simulink library "IO"  (R2024a)
settings: Solver=VariableStepAuto  StartTime=0.0  StopTime=10.0  RelTol=1e-3
values from neighbouring files (symbols this model uses):
  ADCBits = 12.0    [IO.sldd]
  DigitalPolarity : value not decoded    [IO.sldd]
  Vref = 5.0    [IO.sldd]
undefined symbols (not defined in the file or in its folder): Bridge, dt, enum2Raptor, H, raptor_xcp_function
libraries: Raptor_lib x118, Utilities x27, Cooling x1
(part 2 of 4)

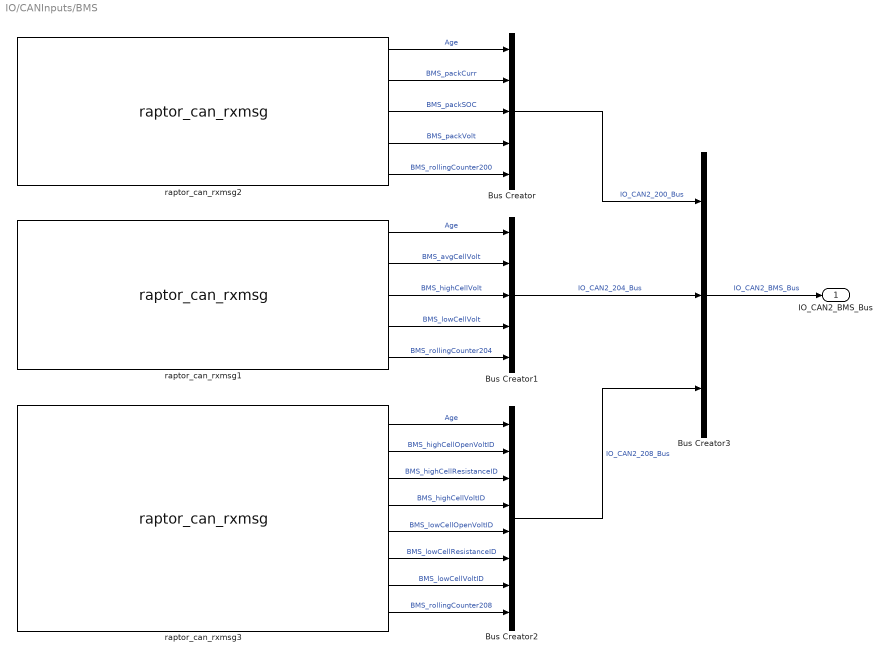
== system IO/CANInputs/BMS ==
  Bus Creator : BusCreator  Inputs=5
  Bus Creator1 : BusCreator  Inputs=5
  Bus Creator2 : BusCreator  Inputs=8
  Bus Creator3 : BusCreator  Inputs=3
  raptor_can_rxmsg1 : Raptor_lib/CAN/raptor_can_rxmsg  canDefinition=struct('dbcFile', 'raptor_CAN2.dbc','message', 'BMS_204','comment', '','signals', {{'BMS_avgCellVolt','BMS_highCellVolt','BMS_lowCellVolt','BMS_rollingCounter204'}},'enabled', [ 1 1 1 1;],'scaled', [ 1 1 1 1;],'canBus', '''CAN2''','messageID', [ 204;],'idMask', [ 536870911;],'payloadMask', [],'payloadValue', [],'period', [ 0;],'mailbox', '''''','queueSize', [ 1;],'label', [ 1;],'ver', [ 2;],'showID', [ 0;],'showRaw', [ 0;],'showRawMsg', [ 0;],'useStartVals', [ 0;],'extendedId', [ 0;],'showAge', [ 1;],'useSimFunc', [ 0;],'sim_func_name', '''''','fill', [ 0;],'editID', [ 0;],'signalOrder', [ 1;],'signalAscDes', [ 1;],'msgLength', [ 8;])  canBus='CAN2'  mailbox=''  payloadMask=[]  payloadValue=[]  idMask=hex2dec('1FFFFFFF')  queueSize=1  showID=0  label=1  fill=0  id=204  showRaw=0  showAge=1  signalOrder=1  signalInfo={{struct('Name', 'BMS_rollingCounter204','StartBit', [ 0;],'SignalSize', [ 8;],'ByteOrder', 'LittleEndian','ValueType', 'UNSIGNED','Class', 'uint8','Signed', [ 0;],'Factor', [ 1;],'Offset', [ 0;],'Min', [ 0;],'Max', [ 255;],'Units', '','StartVal', [ 0;],'Comment', 'Increments once every 100ms (max value is 255 and rolls over). Can be used to ensure data is updating','Multiplexed', [ 0;],'Multiplexor', [ 0;],'MultiplexMode_Min', [],'MultiplexMode_Max', []),struct('Name', 'BMS_lowCellVolt','StartBit', [ 16;],'SignalSize', [ 16;],'ByteOrder', 'LittleEndian','ValueType', 'SIGNED','Class', 'int16','Signed', [ 1;],'Factor', [ 0.0001;],'Offset', [ 0;],'Min', [ -3.2768;],'Max', [ 3.2767;],'Units', 'V','StartVal', [ 0;],'Comment', 'This is the voltage of the lowest measured cell in the battery pack','Multiplexed', [ 0;],'Multiplexor', [ 0;],'MultiplexMode_Min', [],'MultiplexMode_Max', []),struct('Name', 'BMS_highCellVolt','StartBit', [ 32;],'SignalSize', [ 16;],'ByteOrder', 'LittleEndian','ValueType', 'SIGNED','Class', 'int16','Signed', [ 1;],'Factor', [ 0.0001;],'Offset', [ 0;],'Min', [ -3.2768;],'Max', [ 3.2767;],'Units', 'V','StartVal', [ 0;],'Comment', 'This is the voltage of the highest measured cell in the battery pack','Multiplexed', [ 0;],'Multiplexor', [ 0;],'MultiplexMode_Min', [],'MultiplexMode_Max', []),struct('Name', 'BMS_avgCellVolt','StartBit', [ 48;],'SignalSize', [ 16;],'ByteOrder', 'LittleEndian','ValueType', 'SIGNED','Class', 'int16','Signed', [ 1;],'Factor', [ 0.0001;],'Offset', [ 0;],'Min', [ -3.2768;],'Max', [ 3.2767;],'Units', 'V','StartVal', [ 0;],'Comment', 'This is the voltage of the average measured cell in the battery pack','Multiplexed', [ 0;],'Multiplexor', [ 0;],'MultiplexMode_Min', [],'MultiplexMode_Max', [])}}  showRawMsg=0  useSimFunc=0  sim_func_name=''  useStartVals=0  extendedId=0
      settings: SourceProductName=Raptor
  raptor_can_rxmsg2 : Raptor_lib/CAN/raptor_can_rxmsg  canDefinition=struct('dbcFile', 'raptor_CAN2.dbc','message', 'BMS_200','comment', '','signals', {{'BMS_packCurr','BMS_packSOC','BMS_packVolt','BMS_rollingCounter200'}},'enabled', [ 1 1 1 1;],'scaled', [ 1 1 1 1;],'canBus', '''CAN2''','messageID', [ 200;],'idMask', [ 536870911;],'payloadMask', [],'payloadValue', [],'period', [ 0;],'mailbox', '''''','queueSize', [ 1;],'label', [ 1;],'ver', [ 2;],'showID', [ 0;],'showRaw', [ 0;],'showRawMsg', [ 0;],'useStartVals', [ 0;],'extendedId', [ 0;],'showAge', [ 1;],'useSimFunc', [ 0;],'sim_func_name', '''''','fill', [ 0;],'editID', [ 0;],'signalOrder', [ 1;],'signalAscDes', [ 1;],'msgLength', [ 8;])  canBus='CAN2'  mailbox=''  payloadMask=[]  payloadValue=[]  idMask=hex2dec('1FFFFFFF')  queueSize=1  showID=0  label=1  fill=0  id=200  showRaw=0  showAge=1  signalOrder=1  signalInfo={{struct('Name', 'BMS_rollingCounter200','StartBit', [ 0;],'SignalSize', [ 8;],'ByteOrder', 'LittleEndian','ValueType', 'UNSIGNED','Class', 'uint8','Signed', [ 0;],'Factor', [ 1;],'Offset', [ 0;],'Min', [ 0;],'Max', [ 255;],'Units', '','StartVal', [ 0;],'Comment', 'Increments once every 100ms (max value is 255 and rolls over). Can be used to ensure data is updating','Multiplexed', [ 0;],'Multiplexor', [ 0;],'MultiplexMode_Min', [],'MultiplexMode_Max', []),struct('Name', 'BMS_packVolt','StartBit', [ 32;],'SignalSize', [ 16;],'ByteOrder', 'LittleEndian','ValueType', 'SIGNED','Class', 'int16','Signed', [ 1;],'Factor', [ 0.1;],'Offset', [ 0;],'Min', [ -3276.8;],'Max', [ 3276.7;],'Units', 'V','StartVal', [ 0;],'Comment', 'This is the instantaneous total pack voltage value','Multiplexed', [ 0;],'Multiplexor', [ 0;],'MultiplexMode_Min', [],'MultiplexMode_Max', []),struct('Name', 'BMS_packSOC','StartBit', [ 48;],'SignalSize', [ 8;],'ByteOrder', 'LittleEndian','ValueType', 'SIGNED','Class', 'int8','Signed', [ 1;],'Factor', [ 0.5;],'Offset', [ 0;],'Min', [ 0;],'Max', [ 100;],'Units', '%','StartVal', [ 0;],'Comment', 'This is the pack State of Charge','Multiplexed', [ 0;],'Multiplexor', [ 0;],'MultiplexMode_Min', [],'MultiplexMode_Max', []),struct('Name', 'BMS_packCurr','StartBit', [ 16;],'SignalSize', [ 16;],'ByteOrder', 'LittleEndian','ValueType', 'SIGNED','Class', 'int16','Signed', [ 1;],'Factor', [ 0.1;],'Offset', [ 0;],'Min', [ -3276.8;],'Max', [ 3276.7;],'Units', 'A','StartVal', [ 0;],'Comment', 'This is the current pack amperage value for the battery pack. This will report a constant 0 if no current sensor is selected','Multiplexed', [ 0;],'Multiplexor', [ 0;],'MultiplexMode_Min', [],'MultiplexMode_Max', [])}}  showRawMsg=0  useSimFunc=0  sim_func_name=''  useStartVals=0  extendedId=0
      settings: SourceProductName=Raptor
  raptor_can_rxmsg3 : Raptor_lib/CAN/raptor_can_rxmsg  canDefinition=struct('dbcFile', 'raptor_CAN2.dbc','message', 'BMS_208','comment', '','signals', {{'BMS_highCellOpenVoltID','BMS_highCellResistanceID','BMS_highCellVoltID','BMS_lowCellOpenVoltID','BMS_lowCellResistanceID','BMS_lowCellVoltID','BMS_rollingCounter208'}},'enabled', [ 1 1 1 1 1 1 1;],'scaled', [ 1 1 1 1 1 1 1;],'canBus', '''CAN2''','messageID', [ 208;],'idMask', [ 536870911;],'payloadMask', [],'payloadValue', [],'period', [ 0;],'mailbox', '''''','queueSize', [ 1;],'label', [ 1;],'ver', [ 2;],'showID', [ 0;],'showRaw', [ 0;],'showRawMsg', [ 0;],'useStartVals', [ 0;],'extendedId', [ 0;],'showAge', [ 1;],'useSimFunc', [ 0;],'sim_func_name', '''''','fill', [ 0;],'editID', [ 0;],'signalOrder', [ 1;],'signalAscDes', [ 1;],'msgLength', [ 8;])  canBus='CAN2'  mailbox=''  payloadMask=[]  payloadValue=[]  idMask=hex2dec('1FFFFFFF')  queueSize=1  showID=0  label=1  fill=0  id=208  showRaw=0  showAge=1  signalOrder=1  signalInfo={{struct('Name', 'BMS_rollingCounter208','StartBit', [ 0;],'SignalSize', [ 8;],'ByteOrder', 'LittleEndian','ValueType', 'UNSIGNED','Class', 'uint8','Signed', [ 0;],'Factor', [ 1;],'Offset', [ 0;],'Min', [ 0;],'Max', [ 255;],'Units', '','StartVal', [ 0;],'Comment', 'Increments once every 100ms (max value is 255 and rolls over). Can be used to ensure data is updating','Multiplexed', [ 0;],'Multiplexor', [ 0;],'MultiplexMode_Min', [],'MultiplexMode_Max', []),struct('Name', 'BMS_lowCellVoltID','StartBit', [ 8;],'SignalSize', [ 8;],'ByteOrder', 'LittleEndian','ValueType', 'UNSIGNED','Class', 'uint8','Signed', [ 0;],'Factor', [ 1;],'Offset', [ 0;],'Min', [ 1;],'Max', [ 180;],'Units', '','StartVal', [ 0;],'Comment', 'This value is the ID of the lowest cell voltage measured by the BMS. The value is 1 based (valid range: 1-180)','Multiplexed', [ 0;],'Multiplexor', [ 0;],'MultiplexMode_Min', [],'MultiplexMode_Max', []),struct('Name', 'BMS_lowCellResistanceID','StartBit', [ 40;],'SignalSize', [ 8;],'ByteOrder', 'LittleEndian','ValueType', 'UNSIGNED','Class', 'uint8','Signed', [ 0;],'Factor', [ 1;],'Offset', [ 0;],'Min', [ 1;],'Max', [ 180;],'Units', '','StartVal', [ 0;],'Comment', 'This value is the ID of the lowest cell resistance measured by the BMS. The value is 1 based (valid range: 1-180)','Multiplexed', [ 0;],'Multiplexor', [ 0;],'MultiplexMode_Min', [],'MultiplexMode_Max', []),struct('Name', 'BMS_lowCellOpenVoltID','StartBit', [ 24;],'SignalSize', [ 8;],'ByteOrder', 'LittleEndian','ValueType', 'UNSIGNED','Class', 'uint8','Signed', [ 0;],'Factor', [ 1;],'Offset', [ 0;],'Min', [ 1;],'Max', [ 180;],'Units', '','StartVal', [ 0;],'Comment', 'This value is the ID of the lowest cell open (sitting) voltage measured by the BMS. The value is 1 based (valid range: 1-180)','Multiplexed', [ 0;],'Multiplexor', [ 0;],'MultiplexMode_Min', [],'MultiplexMode_Max', []),struct('Name', 'BMS_highCellVoltID','StartBit', [ 16;],'SignalSize', [ 8;],'ByteOrder', 'LittleEndian','ValueType', 'UNSIGNED','Class', 'uint8','Signed', [ 0;],'Factor', [ 1;],'Offset', [ 0;],'Min', [ 1;],'Max', [ 180;],'Units', '','StartVal', [ 0;],'Comment', 'This value is the ID of the highest cell voltage measured by the BMS. The value is 1 based (valid range: 1-180)','Multiplexed', [ 0;],'Multiplexor', [ 0;],'MultiplexMode_Min', [],'MultiplexMode_Max', []),struct('Name', 'BMS_highCellResistanceID','StartBit', [ 48;],'SignalSize', [ 8;],'ByteOrder', 'LittleEndian','ValueType', 'UNSIGNED','Class', 'uint8','Signed', [ 0;],'Factor', [ 1;],'Offset', [ 0;],'Min', [ 1;],'Max', [ 180;],'Units', '','StartVal', [ 0;],'Comment', 'This value is the ID of the highest cell resistance measured by the BMS. The value is 1 based (valid range: 1-180)','Multiplexed', [ 0;],'Multiplexor', [ 0;],'MultiplexMode_Min', [],'MultiplexMode_Max', []),struct('Name', 'BMS_highCellOpenVoltID','StartBit', [ 32;],'SignalSize', [ 8;],'ByteOrder', 'LittleEndian','ValueType', 'UNSIGNED','Class', 'uint8','Signed', [ 0;],'Factor', [ 1;],'Offset', [ 0;],'Min', [ 1;],'Max', [ 180;],'Units', '','StartVal', [ 0;],'Comment', 'This value is the ID of the highest cell open (sitting) voltage measured by the BMS. The value is 1 based (valid range: 1-180)','Multiplexed', [ 0;],'Multiplexor', [ 0;],'MultiplexMode_Min', [],'MultiplexMode_Max', [])}}  showRawMsg=0  useSimFunc=0  sim_func_name=''  useStartVals=0  extendedId=0
      settings: SourceProductName=Raptor
  IO_CAN2_BMS_Bus : Outport
  wires:
  Bus Creator3/1 -> IO_CAN2_BMS_Bus/1  "IO_CAN2_BMS_Bus"
  Bus Creator2/1 -> Bus Creator3/3  "IO_CAN2_208_Bus"
  Bus Creator/1 -> Bus Creator3/1  "IO_CAN2_200_Bus"
  Bus Creator1/1 -> Bus Creator3/2  "IO_CAN2_204_Bus"
  raptor_can_rxmsg3/8 -> Bus Creator2/8  "BMS_rollingCounter208"
  raptor_can_rxmsg3/7 -> Bus Creator2/7  "BMS_lowCellVoltID"
  raptor_can_rxmsg3/6 -> Bus Creator2/6  "BMS_lowCellResistanceID"
  raptor_can_rxmsg3/5 -> Bus Creator2/5  "BMS_lowCellOpenVoltID"
  raptor_can_rxmsg3/4 -> Bus Creator2/4  "BMS_highCellVoltID"
  raptor_can_rxmsg3/3 -> Bus Creator2/3  "BMS_highCellResistanceID"
  raptor_can_rxmsg3/2 -> Bus Creator2/2  "BMS_highCellOpenVoltID"
  raptor_can_rxmsg3/1 -> Bus Creator2/1  "Age"
  raptor_can_rxmsg1/5 -> Bus Creator1/5  "BMS_rollingCounter204"
  raptor_can_rxmsg1/4 -> Bus Creator1/4  "BMS_lowCellVolt"
  raptor_can_rxmsg1/3 -> Bus Creator1/3  "BMS_highCellVolt"
  raptor_can_rxmsg1/2 -> Bus Creator1/2  "BMS_avgCellVolt"
  raptor_can_rxmsg1/1 -> Bus Creator1/1  "Age"
  raptor_can_rxmsg2/5 -> Bus Creator/5  "BMS_rollingCounter200"
  raptor_can_rxmsg2/4 -> Bus Creator/4  "BMS_packVolt"
  raptor_can_rxmsg2/3 -> Bus Creator/3  "BMS_packSOC"
  raptor_can_rxmsg2/2 -> Bus Creator/2  "BMS_packCurr"
  raptor_can_rxmsg2/1 -> Bus Creator/1  "Age"

== system IO/CANInputs/DCDC ==
  Bus Creator : BusCreator  Inputs=19
  Bus Creator1 : BusCreator  Inputs=1
  raptor_can_rxmsg : Raptor_lib/CAN/raptor_can_rxmsg  canDefinition=struct('dbcFile', 'raptor_CAN1.dbc','message', 'DCDC_1801D08F','comment', '','signals', {{'DCDC_canError','DCDC_currentOutput','DCDC_fanControl1','DCDC_fanControl2','DCDC_hardwareFault','DCDC_hvilError','DCDC_inputOverVoltage','DCDC_inputUnderVoltage','DCDC_outputOverCurrent','DCDC_outputOverVoltage','DCDC_outputUnderVoltage','DCDC_overTempError','DCDC_ready','DCDC_shutOffError','DCDC_status','DCDC_tempWarning','DCDC_temperature','DCDC_voltageOutput'}},'enabled', [ 1 1 1 1 1 1 1 1 1 1 1 1 1 1 1 1 1 1;],'scaled', [ 1 1 1 1 1 1 1 1 1 1 1 1 1 1 1 1 1 1;],'canBus', '''CAN1''','messageID', [ 402772111;],'idMask', [ 536870911;],'payloadMask', [],'payloadValue', [],'period', [ 0;],'mailbox', '''''','queueSize', [ 1;],'label', [ 1;],'ver', [ 2;],'showID', [ 0;],'showRaw', [ 0;],'showRawMsg', [ 0;],'useStartVals', [ 0;],'extendedId', [ 1;],'showAge', [ 1;],'useSimFunc', [ 0;],'sim_func_name', '''''','fill', [ 0;],'editID', [ 0;],'signalOrder', [ 1;],'signalAscDes', [ 1;],'msgLength', [ 8;])  canBus='CAN1'  mailbox=''  payloadMask=[]  payloadValue=[]  idMask=hex2dec('1FFFFFFF')  queueSize=1  showID=0  label=1  fill=0  id=402772111  showRaw=0  showAge=1  signalOrder=1  signalInfo={{struct('Name', 'DCDC_temperature','StartBit', [ 56;],'SignalSize', [ 16;],'ByteOrder', 'BigEndian','ValueType', 'SIGNED','Class', 'int16','Signed', [ 1;],'Factor', [ 0.1;],'Offset', [ 0;],'Min', [ -3276.8;],'Max', [ 3276.7;],'Units', 'degC','StartVal', [ 0;],'Comment', 'DCDC temperature','Multiplexed', [ 0;],'Multiplexor', [ 0;],'MultiplexMode_Min', [],'MultiplexMode_Max', []),struct('Name', 'DCDC_outputOverCurrent','StartBit', [ 46;],'SignalSize', [ 1;],'ByteOrder', 'LittleEndian','ValueType', 'UNSIGNED','Class', 'uint8','Signed', [ 0;],'Factor', [ 1;],'Offset', [ 0;],'Min', [ 0;],'Max', [ 1;],'Units', '','StartVal', [ 0;],'Comment', 'DCDC output over current; 0: no error, 1: error','Multiplexed', [ 0;],'Multiplexor', [ 0;],'MultiplexMode_Min', [],'MultiplexMode_Max', []),struct('Name', 'DCDC_outputUnderVoltage','StartBit', [ 45;],'SignalSize', [ 1;],'ByteOrder', 'LittleEndian','ValueType', 'UNSIGNED','Class', 'uint8','Signed', [ 0;],'Factor', [ 1;],'Offset', [ 0;],'Min', [ 0;],'Max', [ 1;],'Units', '','StartVal', [ 0;],'Comment', 'DCDC output under voltage; 0: no error, 1: error','Multiplexed', [ 0;],'Multiplexor', [ 0;],'MultiplexMode_Min', [],'MultiplexMode_Max', []),struct('Name', 'DCDC_outputOverVoltage','StartBit', [ 44;],'SignalSize', [ 1;],'ByteOrder', 'LittleEndian','ValueType', 'UNSIGNED','Class', 'uint8','Signed', [ 0;],'Factor', [ 1;],'Offset', [ 0;],'Min', [ 0;],'Max', [ 1;],'Units', '','StartVal', [ 0;],'Comment', 'DCDC output over voltage; 0: no error, 1: error','Multiplexed', [ 0;],'Multiplexor', [ 0;],'MultiplexMode_Min', [],'MultiplexMode_Max', []),struct('Name', 'DCDC_inputUnderVoltage','StartBit', [ 43;],'SignalSize', [ 1;],'ByteOrder', 'LittleEndian','ValueType', 'UNSIGNED','Class', 'uint8','Signed', [ 0;],'Factor', [ 1;],'Offset', [ 0;],'Min', [ 0;],'Max', [ 1;],'Units', '','StartVal', [ 0;],'Comment', 'DCDC input under voltage; 0: no error, 1: error','Multiplexed', [ 0;],'Multiplexor', [ 0;],'MultiplexMode_Min', [],'MultiplexMode_Max', []),struct('Name', 'DCDC_inputOverVoltage','StartBit', [ 42;],'SignalSize', [ 1;],'ByteOrder', 'LittleEndian','ValueType', 'UNSIGNED','Class', 'uint8','Signed', [ 0;],'Factor', [ 1;],'Offset', [ 0;],'Min', [ 0;],'Max', [ 1;],'Units', '','StartVal', [ 0;],'Comment', 'DCDC input over voltage; 0: no error, 1: error','Multiplexed', [ 0;],'Multiplexor', [ 0;],'MultiplexMode_Min', [],'MultiplexMode_Max', []),struct('Name', 'DCDC_overTempError','StartBit', [ 41;],'SignalSize', [ 1;],'ByteOrder', 'LittleEndian','ValueType', 'UNSIGNED','Class', 'uint8','Signed', [ 0;],'Factor', [ 1;],'Offset', [ 0;],'Min', [ 0;],'Max', [ 1;],'Units', '','StartVal', [ 0;],'Comment', 'DCDC over temp error; 0: no error, 1: error','Multiplexed', [ 0;],'Multiplexor', [ 0;],'MultiplexMode_Min', [],'MultiplexMode_Max', []),struct('Name', 'DCDC_tempWarning','StartBit', [ 40;],'SignalSize', [ 1;],'ByteOrder', 'LittleEndian','ValueType', 'UNSIGNED','Class', 'uint8','Signed', [ 0;],'Factor', [ 1;],'Offset', [ 0;],'Min', [ 0;],'Max', [ 1;],'Units', '','StartVal', [ 0;],'Comment', 'DCDC over temp warning; 0: no warning, 1: warning','Multiplexed', [ 0;],'Multiplexor', [ 0;],'MultiplexMode_Min', [],'MultiplexMode_Max', []),struct('Name', 'DCDC_hvilError','StartBit', [ 39;],'SignalSize', [ 1;],'ByteOrder', 'LittleEndian','ValueType', 'UNSIGNED','Class', 'uint8','Signed', [ 0;],'Factor', [ 1;],'Offset', [ 0;],'Min', [ 0;],'Max', [ 1;],'Units', '','StartVal', [ 0;],'Comment', 'High Voltage Interlock error; 0: no error, 1: error','Multiplexed', [ 0;],'Multiplexor', [ 0;],'MultiplexMode_Min', [],'MultiplexMode_Max', []),struct('Name', 'DCDC_fanControl2','StartBit', [ 38;],'SignalSize', [ 1;],'ByteOrder', 'LittleEndian','ValueType', 'UNSIGNED','Class', 'uint8','Signed', [ 0;],'Factor', [ 1;],'Offset', [ 0;],'Min', [ 0;],'Max', [ 1;],'Units', '','StartVal', [ 0;],'Comment', 'DCDC fan control; 0: off, 1: on','Multiplexed', [ 0;],'Multiplexor', [ 0;],'MultiplexMode_Min', [],'MultiplexMode_Max', []),struct('Name', 'DCDC_shutOffError','StartBit', [ 37;],'SignalSize', [ 1;],'ByteOrder', 'LittleEndian','ValueType', 'UNSIGNED','Class', 'uint8','Signed', [ 0;],'Factor', [ 1;],'Offset', [ 0;],'Min', [ 0;],'Max', [ 1;],'Units', '','StartVal', [ 0;],'Comment', 'DCDC shut off error; 0: no error, 1: error','Multiplexed', [ 0;],'Multiplexor', [ 0;],'MultiplexMode_Min', [],'MultiplexMode_Max', []),struct('Name', 'DCDC_fanControl1','StartBit', [ 36;],'SignalSize', [ 1;],'ByteOrder', 'LittleEndian','ValueType', 'UNSIGNED','Class', 'uint8','Signed', [ 0;],'Factor', [ 1;],'Offset', [ 0;],'Min', [ 0;],'Max', [ 1;],'Units', '','StartVal', [ 0;],'Comment', '','Multiplexed', [ 0;],'Multiplexor', [ 0;],'MultiplexMode_Min', [],'MultiplexMode_Max', []),struct('Name', 'DCDC_canError','StartBit', [ 35;],'SignalSize', [ 1;],'ByteOrder', 'LittleEndian','ValueType', 'UNSIGNED','Class', 'uint8','Signed', [ 0;],'Factor', [ 1;],'Offset', [ 0;],'Min', [ 0;],'Max', [ 1;],'Units', '','StartVal', [ 0;],'Comment', 'DCDC CAN error; 0: no error, 1: error','Multiplexed', [ 0;],'Multiplexor', [ 0;],'MultiplexMode_Min', [],'MultiplexMode_Max', []),struct('Name', 'DCDC_hardwareFault','StartBit', [ 34;],'SignalSize', [ 1;],'ByteOrder', 'LittleEndian','ValueType', 'UNSIGNED','Class', 'uint8','Signed', [ 0;],'Factor', [ 1;],'Offset', [ 0;],'Min', [ 0;],'Max', [ 1;],'Units', '','StartVal', [ 0;],'Comment', 'DCDC hardware error; 0: no error, 1: error','Multiplexed', [ 0;],'Multiplexor', [ 0;],'MultiplexMode_Min', [],'MultiplexMode_Max', []),struct('Name', 'DCDC_status','StartBit', [ 33;],'SignalSize', [ 1;],'ByteOrder', 'LittleEndian','ValueType', 'UNSIGNED','Class', 'uint8','Signed', [ 0;],'Factor', [ 1;],'Offset', [ 0;],'Min', [ 0;],'Max', [ 1;],'Units', '','StartVal', [ 0;],'Comment', 'DCDC state; 0: stopped, 1: working','Multiplexed', [ 0;],'Multiplexor', [ 0;],'MultiplexMode_Min', [],'MultiplexMode_Max', []),struct('Name', 'DCDC_ready','StartBit', [ 32;],'SignalSize', [ 1;],'ByteOrder', 'LittleEndian','ValueType', 'UNSIGNED','Class', 'uint8','Signed', [ 0;],'Factor', [ 1;],'Offset', [ 0;],'Min', [ 0;],'Max', [ 1;],'Units', '','StartVal', [ 0;],'Comment', 'DCDC initialization status; 0: incomplete, 1: complete','Multiplexed', [ 0;],'Multiplexor', [ 0;],'MultiplexMode_Min', [],'MultiplexMode_Max', []),struct('Name', 'DCDC_currentOutput','StartBit', [ 24;],'SignalSize', [ 16;],'ByteOrder', 'BigEndian','ValueType', 'UNSIGNED','Class', 'uint16','Signed', [ 0;],'Factor', [ 0.1;],'Offset', [ 0;],'Min', [ 0;],'Max', [ 6553.5;],'Units', 'A','StartVal', [ 0;],'Comment', 'DCDC output current','Multiplexed', [ 0;],'Multiplexor', [ 0;],'MultiplexMode_Min', [],'MultiplexMode_Max', []),struct('Name', 'DCDC_voltageOutput','StartBit', [ 8;],'SignalSize', [ 16;],'ByteOrder', 'BigEndian','ValueType', 'UNSIGNED','Class', 'uint16','Signed', [ 0;],'Factor', [ 0.1;],'Offset', [ 0;],'Min', [ 0;],'Max', [ 6553.5;],'Units', 'V','StartVal', [ 0;],'Comment', 'DCDC output voltage','Multiplexed', [ 0;],'Multiplexor', [ 0;],'MultiplexMode_Min', [],'MultiplexMode_Max', [])}}  showRawMsg=0  useSimFunc=0  sim_func_name=''  useStartVals=0  extendedId=1
      settings: SourceProductName=Raptor
  IO_CAN1_DCDC_Bus : Outport
  wires:
  raptor_can_rxmsg/10 -> Bus Creator/10  "DCDC_outputOverCurrent"
  raptor_can_rxmsg/8 -> Bus Creator/8  "DCDC_inputOverVoltage"
  raptor_can_rxmsg/7 -> Bus Creator/7  "DCDC_hvilError"
  Bus Creator1/1 -> IO_CAN1_DCDC_Bus/1  "IO_CAN1_DCDC_Bus"
  Bus Creator/1 -> Bus Creator1/1  "IO_CAN1_402772111_Bus"
  raptor_can_rxmsg/19 -> Bus Creator/19  "DCDC_voltageOutput"
  raptor_can_rxmsg/18 -> Bus Creator/18  "DCDC_temperature"
  raptor_can_rxmsg/17 -> Bus Creator/17  "DCDC_tempWarning"
  raptor_can_rxmsg/16 -> Bus Creator/16  "DCDC_status"
  raptor_can_rxmsg/15 -> Bus Creator/15  "DCDC_shutOffError"
  raptor_can_rxmsg/14 -> Bus Creator/14  "DCDC_ready"
  raptor_can_rxmsg/13 -> Bus Creator/13  "DCDC_overTempError"
  raptor_can_rxmsg/12 -> Bus Creator/12  "DCDC_outputUnderVoltage"
  raptor_can_rxmsg/11 -> Bus Creator/11  "DCDC_outputOverVoltage"
  raptor_can_rxmsg/9 -> Bus Creator/9  "DCDC_inputUnderVoltage"
  raptor_can_rxmsg/6 -> Bus Creator/6  "DCDC_hardwareFault"
  raptor_can_rxmsg/5 -> Bus Creator/5  "DCDC_fanControl2"
  raptor_can_rxmsg/4 -> Bus Creator/4  "DCDC_fanControl1"
  raptor_can_rxmsg/3 -> Bus Creator/3  "DCDC_currentOutput"
  raptor_can_rxmsg/2 -> Bus Creator/2  "DCDC_canError"
  raptor_can_rxmsg/1 -> Bus Creator/1  "Age"

== system IO/CANInputs/LWS ==
  Bus Creator : BusCreator  Inputs=6
  Bus Creator1 : BusCreator  Inputs=1
  raptor_can_rxmsg2 : Raptor_lib/CAN/raptor_can_rxmsg  canDefinition=struct('dbcFile', 'raptor_CAN1.dbc','message', 'LWS_688','comment', '','signals', {{'LWS_angle','LWS_cal','LWS_ok','LWS_speed','LWS_trim'}},'enabled', [ 1 1 1 1 1;],'scaled', [ 1 1 1 1 1;],'canBus', '''CAN1''','messageID', [ 688;],'idMask', [ 536870911;],'payloadMask', [],'payloadValue', [],'period', [ 0;],'mailbox', '''''','queueSize', [ 1;],'label', [ 1;],'ver', [ 2;],'showID', [ 0;],'showRaw', [ 0;],'showRawMsg', [ 0;],'useStartVals', [ 0;],'extendedId', [ 0;],'showAge', [ 1;],'useSimFunc', [ 0;],'sim_func_name', '''''','fill', [ 0;],'editID', [ 0;],'signalOrder', [ 1;],'signalAscDes', [ 1;],'msgLength', [ 8;])  canBus='CAN1'  mailbox=''  payloadMask=[]  payloadValue=[]  idMask=hex2dec('1FFFFFFF')  queueSize=1  showID=0  label=1  fill=0  id=688  showRaw=0  showAge=1  signalOrder=1  signalInfo={{struct('Name', 'LWS_trim','StartBit', [ 26;],'SignalSize', [ 1;],'ByteOrder', 'LittleEndian','ValueType', 'UNSIGNED','Class', 'uint8','Signed', [ 0;],'Factor', [ 1;],'Offset', [ 0;],'Min', [ 0;],'Max', [ 1;],'Units', '','StartVal', [ 0;],'Comment', 'Consult truth table','Multiplexed', [ 0;],'Multiplexor', [ 0;],'MultiplexMode_Min', [],'MultiplexMode_Max', []),struct('Name', 'LWS_cal','StartBit', [ 25;],'SignalSize', [ 1;],'ByteOrder', 'LittleEndian','ValueType', 'UNSIGNED','Class', 'uint8','Signed', [ 0;],'Factor', [ 1;],'Offset', [ 0;],'Min', [ 0;],'Max', [ 1;],'Units', '','StartVal', [ 0;],'Comment', 'Consult truth table','Multiplexed', [ 0;],'Multiplexor', [ 0;],'MultiplexMode_Min', [],'MultiplexMode_Max', []),struct('Name', 'LWS_ok','StartBit', [ 24;],'SignalSize', [ 1;],'ByteOrder', 'LittleEndian','ValueType', 'UNSIGNED','Class', 'uint8','Signed', [ 0;],'Factor', [ 1;],'Offset', [ 0;],'Min', [ 0;],'Max', [ 1;],'Units', '','StartVal', [ 0;],'Comment', 'Consult truth table','Multiplexed', [ 0;],'Multiplexor', [ 0;],'MultiplexMode_Min', [],'MultiplexMode_Max', []),struct('Name', 'LWS_speed','StartBit', [ 16;],'SignalSize', [ 8;],'ByteOrder', 'LittleEndian','ValueType', 'UNSIGNED','Class', 'uint8','Signed', [ 0;],'Factor', [ 4;],'Offset', [ 0;],'Min', [ 0;],'Max', [ 1020;],'Units', 'deg/s','StartVal', [ 0;],'Comment', 'Angular Speed','Multiplexed', [ 0;],'Multiplexor', [ 0;],'MultiplexMode_Min', [],'MultiplexMode_Max', []),struct('Name', 'LWS_angle','StartBit', [ 0;],'SignalSize', [ 16;],'ByteOrder', 'LittleEndian','ValueType', 'SIGNED','Class', 'int16','Signed', [ 1;],'Factor', [ 0.1;],'Offset', [ 0;],'Min', [ -3276.8;],'Max', [ 3276.7;],'Units', 'deg','StartVal', [ 0;],'Comment', 'Steering Wheel Angle','Multiplexed', [ 0;],'Multiplexor', [ 0;],'MultiplexMode_Min', [],'MultiplexMode_Max', [])}}  showRawMsg=0  useSimFunc=0  sim_func_name=''  useStartVals=0  extendedId=0
      settings: SourceProductName=Raptor
  IO_CAN1_LWS_Bus : Outport
  wires:
  Bus Creator1/1 -> IO_CAN1_LWS_Bus/1  "IO_CAN1_LWS_Bus"
  Bus Creator/1 -> Bus Creator1/1  "IO_CAN1_688_Bus"
  raptor_can_rxmsg2/6 -> Bus Creator/6  "LWS_trim"
  raptor_can_rxmsg2/5 -> Bus Creator/5  "LWS_speed"
  raptor_can_rxmsg2/4 -> Bus Creator/4  "LWS_ok"
  raptor_can_rxmsg2/3 -> Bus Creator/3  "LWS_cal"
  raptor_can_rxmsg2/2 -> Bus Creator/2  "LWS_angle"
  raptor_can_rxmsg2/1 -> Bus Creator/1  "Age"

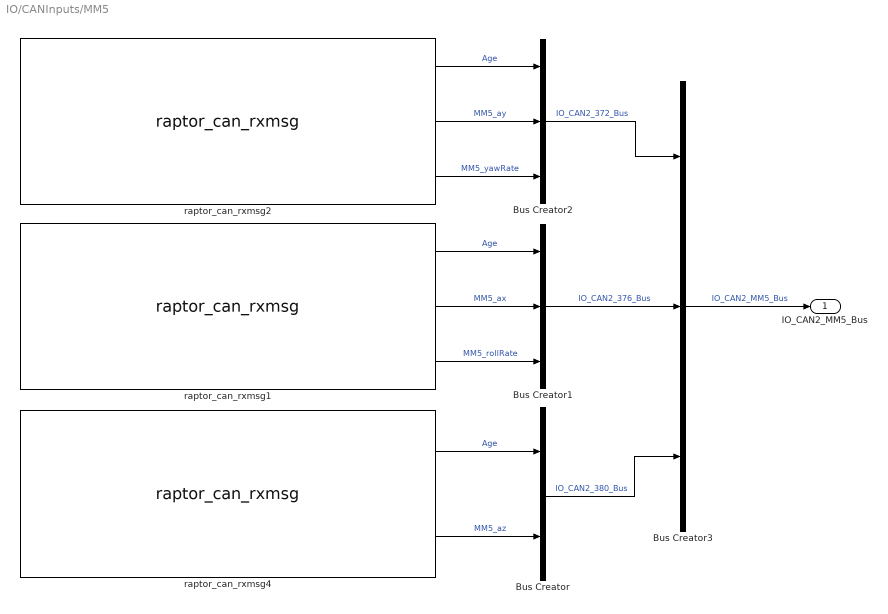
== system IO/CANInputs/MM5 ==
  Bus Creator : BusCreator  Inputs=2
  Bus Creator1 : BusCreator  Inputs=3
  Bus Creator2 : BusCreator  Inputs=3
  Bus Creator3 : BusCreator  Inputs=3
  raptor_can_rxmsg1 : Raptor_lib/CAN/raptor_can_rxmsg  canDefinition=struct('dbcFile', 'raptor_CAN2.dbc','message', 'MM5_376','comment', '','signals', {{'MM5_ax','MM5_rollRate'}},'enabled', [ 1 1;],'scaled', [ 1 1;],'canBus', '''CAN2''','messageID', [ 376;],'idMask', [ 536870911;],'payloadMask', [],'payloadValue', [],'period', [ 0;],'mailbox', '''''','queueSize', [ 1;],'label', [ 1;],'ver', [ 2;],'showID', [ 0;],'showRaw', [ 0;],'showRawMsg', [ 0;],'useStartVals', [ 0;],'extendedId', [ 0;],'showAge', [ 1;],'useSimFunc', [ 0;],'sim_func_name', '''''','fill', [ 0;],'editID', [ 0;],'signalOrder', [ 1;],'signalAscDes', [ 1;],'msgLength', [ 8;])  canBus='CAN2'  mailbox=''  payloadMask=[]  payloadValue=[]  idMask=hex2dec('1FFFFFFF')  queueSize=1  showID=0  label=1  fill=0  id=376  showRaw=0  showAge=1  signalOrder=1  signalInfo={{struct('Name', 'MM5_rollRate','StartBit', [ 0;],'SignalSize', [ 16;],'ByteOrder', 'LittleEndian','ValueType', 'UNSIGNED','Class', 'uint16','Signed', [ 0;],'Factor', [ -0.005;],'Offset', [ 163.9;],'Min', [ -163.775;],'Max', [ 163.9;],'Units', 'deg/s','StartVal', [ 0;],'Comment', 'Roll Rate','Multiplexed', [ 0;],'Multiplexor', [ 0;],'MultiplexMode_Min', [],'MultiplexMode_Max', []),struct('Name', 'MM5_ax','StartBit', [ 32;],'SignalSize', [ 16;],'ByteOrder', 'LittleEndian','ValueType', 'UNSIGNED','Class', 'uint16','Signed', [ 0;],'Factor', [ -0.0001274;],'Offset', [ 4.1746;],'Min', [ -4.1746;],'Max', [ 4.1746;],'Units', 'g','StartVal', [ 0;],'Comment', 'Acceleration X Axis','Multiplexed', [ 0;],'Multiplexor', [ 0;],'MultiplexMode_Min', [],'MultiplexMode_Max', [])}}  showRawMsg=0  useSimFunc=0  sim_func_name=''  useStartVals=0  extendedId=0
      settings: SourceProductName=Raptor
  raptor_can_rxmsg2 : Raptor_lib/CAN/raptor_can_rxmsg  canDefinition=struct('dbcFile', 'raptor_CAN2.dbc','message', 'MM5_372','comment', '','signals', {{'MM5_ay','MM5_yawRate'}},'enabled', [ 1 1;],'scaled', [ 1 1;],'canBus', '''CAN2''','messageID', [ 372;],'idMask', [ 536870911;],'payloadMask', [],'payloadValue', [],'period', [ 0;],'mailbox', '''''','queueSize', [ 1;],'label', [ 1;],'ver', [ 2;],'showID', [ 0;],'showRaw', [ 0;],'showRawMsg', [ 0;],'useStartVals', [ 0;],'extendedId', [ 0;],'showAge', [ 1;],'useSimFunc', [ 0;],'sim_func_name', '''''','fill', [ 0;],'editID', [ 0;],'signalOrder', [ 1;],'signalAscDes', [ 1;],'msgLength', [ 8;])  canBus='CAN2'  mailbox=''  payloadMask=[]  payloadValue=[]  idMask=hex2dec('1FFFFFFF')  queueSize=1  showID=0  label=1  fill=0  id=372  showRaw=0  showAge=1  signalOrder=1  signalInfo={{struct('Name', 'MM5_yawRate','StartBit', [ 0;],'SignalSize', [ 16;],'ByteOrder', 'LittleEndian','ValueType', 'UNSIGNED','Class', 'uint16','Signed', [ 0;],'Factor', [ 0.005;],'Offset', [ -163.9;],'Min', [ -163.9;],'Max', [ 163.775;],'Units', 'deg/s','StartVal', [ 0;],'Comment', 'Yaw Rate','Multiplexed', [ 0;],'Multiplexor', [ 0;],'MultiplexMode_Min', [],'MultiplexMode_Max', []),struct('Name', 'MM5_ay','StartBit', [ 32;],'SignalSize', [ 16;],'ByteOrder', 'LittleEndian','ValueType', 'UNSIGNED','Class', 'uint16','Signed', [ 0;],'Factor', [ -0.0001274;],'Offset', [ 4.1746;],'Min', [ -4.1746;],'Max', [ 4.1746;],'Units', 'g','StartVal', [ 0;],'Comment', 'Acceleration Y Axis','Multiplexed', [ 0;],'Multiplexor', [ 0;],'MultiplexMode_Min', [],'MultiplexMode_Max', [])}}  showRawMsg=0  useSimFunc=0  sim_func_name=''  useStartVals=0  extendedId=0
      settings: SourceProductName=Raptor
  raptor_can_rxmsg4 : Raptor_lib/CAN/raptor_can_rxmsg  canDefinition=struct('dbcFile', 'raptor_CAN2.dbc','message', 'MM5_380','comment', '','signals', {{'MM5_az'}},'enabled', [ 1;],'scaled', [ 1;],'canBus', '''CAN2''','messageID', [ 380;],'idMask', [ 536870911;],'payloadMask', [],'payloadValue', [],'period', [ 0;],'mailbox', '''''','queueSize', [ 1;],'label', [ 1;],'ver', [ 2;],'showID', [ 0;],'showRaw', [ 0;],'showRawMsg', [ 0;],'useStartVals', [ 0;],'extendedId', [ 0;],'showAge', [ 1;],'useSimFunc', [ 0;],'sim_func_name', '''''','fill', [ 0;],'editID', [ 0;],'signalOrder', [ 1;],'signalAscDes', [ 1;],'msgLength', [ 8;])  canBus='CAN2'  mailbox=''  payloadMask=[]  payloadValue=[]  idMask=hex2dec('1FFFFFFF')  queueSize=1  showID=0  label=1  fill=0  id=380  showRaw=0  showAge=1  signalOrder=1  signalInfo={{struct('Name', 'MM5_az','StartBit', [ 32;],'SignalSize', [ 16;],'ByteOrder', 'LittleEndian','ValueType', 'UNSIGNED','Class', 'uint16','Signed', [ 0;],'Factor', [ -0.0001274;],'Offset', [ 4.1746;],'Min', [ -4.1746;],'Max', [ 4.1746;],'Units', 'g','StartVal', [ 0;],'Comment', 'Acceleration Z Axis','Multiplexed', [ 0;],'Multiplexor', [ 0;],'MultiplexMode_Min', [],'MultiplexMode_Max', [])}}  showRawMsg=0  useSimFunc=0  sim_func_name=''  useStartVals=0  extendedId=0
      settings: SourceProductName=Raptor
  IO_CAN2_MM5_Bus : Outport
  wires:
  Bus Creator3/1 -> IO_CAN2_MM5_Bus/1  "IO_CAN2_MM5_Bus"
  Bus Creator2/1 -> Bus Creator3/1  "IO_CAN2_372_Bus"
  Bus Creator/1 -> Bus Creator3/3  "IO_CAN2_380_Bus"
  Bus Creator1/1 -> Bus Creator3/2  "IO_CAN2_376_Bus"
  raptor_can_rxmsg2/3 -> Bus Creator2/3  "MM5_yawRate"
  raptor_can_rxmsg2/1 -> Bus Creator2/1  "Age"
  raptor_can_rxmsg2/2 -> Bus Creator2/2  "MM5_ay"
  raptor_can_rxmsg1/3 -> Bus Creator1/3  "MM5_rollRate"
  raptor_can_rxmsg1/1 -> Bus Creator1/1  "Age"
  raptor_can_rxmsg1/2 -> Bus Creator1/2  "MM5_ax"
  raptor_can_rxmsg4/2 -> Bus Creator/2  "MM5_az"
  raptor_can_rxmsg4/1 -> Bus Creator/1  "Age"

== system IO/CANInputs/PDM ==
  Out1 : Outport

== system IO/CANInputs/PM100DX ==
  Bus Creator : BusCreator  Inputs=5
  Bus Creator1 : BusCreator  Inputs=3
  Bus Creator2 : BusCreator  Inputs=5
  Bus Creator3 : BusCreator  Inputs=5
  raptor_can_rxmsg : Raptor_lib/CAN/raptor_can_rxmsg  canDefinition=struct('dbcFile', 'raptor_CAN1.dbc','message', 'PM_167','comment', '','signals', {{'PM_dcBusVolt','PM_outputVolt','PM_vabVdVolt','PM_vbcVqVolt'}},'enabled', [ 1 1 1 1;],'scaled', [ 1 1 1 1;],'canBus', '''CAN1''','messageID', [ 167;],'idMask', [ 536870911;],'payloadMask', [],'payloadValue', [],'period', [ 0;],'mailbox', '''''','queueSize', [ 1;],'label', [ 1;],'ver', [ 2;],'showID', [ 0;],'showRaw', [ 0;],'showRawMsg', [ 0;],'useStartVals', [ 0;],'extendedId', [ 0;],'showAge', [ 1;],'useSimFunc', [ 0;],'sim_func_name', '''''','fill', [ 0;],'editID', [ 0;],'signalOrder', [ 1;],'signalAscDes', [ 1;],'msgLength', [ 8;])  canBus='CAN1'  mailbox=''  payloadMask=[]  payloadValue=[]  idMask=hex2dec('1FFFFFFF')  queueSize=1  showID=0  label=1  fill=0  id=167  showRaw=0  showAge=1  signalOrder=1  signalInfo={{struct('Name', 'PM_vbcVqVolt','StartBit', [ 48;],'SignalSize', [ 16;],'ByteOrder', 'LittleEndian','ValueType', 'SIGNED','Class', 'int16','Signed', [ 1;],'Factor', [ 0.1;],'Offset', [ 0;],'Min', [ -3276.8;],'Max', [ 3276.7;],'Units', 'V','StartVal', [ 0;],'Comment', 'Measured value of the voltage between Phase B and Phase C','Multiplexed', [ 0;],'Multiplexor', [ 0;],'MultiplexMode_Min', [],'MultiplexMode_Max', []),struct('Name', 'PM_vabVdVolt','StartBit', [ 32;],'SignalSize', [ 16;],'ByteOrder', 'LittleEndian','ValueType', 'SIGNED','Class', 'int16','Signed', [ 1;],'Factor', [ 0.1;],'Offset', [ 0;],'Min', [ -3276.8;],'Max', [ 3276.7;],'Units', 'V','StartVal', [ 0;],'Comment', 'Measured value of the voltage between Phase A and Phase B','Multiplexed', [ 0;],'Multiplexor', [ 0;],'MultiplexMode_Min', [],'MultiplexMode_Max', []),struct('Name', 'PM_outputVolt','StartBit', [ 16;],'SignalSize', [ 16;],'ByteOrder', 'LittleEndian','ValueType', 'SIGNED','Class', 'int16','Signed', [ 1;],'Factor', [ 0.1;],'Offset', [ 0;],'Min', [ -3276.8;],'Max', [ 3276.7;],'Units', 'V','StartVal', [ 0;],'Comment', 'The calculated value of the output voltage, in peak line-neutral volts','Multiplexed', [ 0;],'Multiplexor', [ 0;],'MultiplexMode_Min', [],'MultiplexMode_Max', []),struct('Name', 'PM_dcBusVolt','StartBit', [ 0;],'SignalSize', [ 16;],'ByteOrder', 'LittleEndian','ValueType', 'SIGNED','Class', 'int16','Signed', [ 1;],'Factor', [ 0.1;],'Offset', [ 0;],'Min', [ -3276.8;],'Max', [ 3276.7;],'Units', 'V','StartVal', [ 0;],'Comment', 'The actual measured value of the DC bus voltage','Multiplexed', [ 0;],'Multiplexor', [ 0;],'MultiplexMode_Min', [],'MultiplexMode_Max', [])}}  showRawMsg=0  useSimFunc=0  sim_func_name=''  useStartVals=0  extendedId=0
      settings: SourceProductName=Raptor
  raptor_can_rxmsg1 : Raptor_lib/CAN/raptor_can_rxmsg  canDefinition=struct('dbcFile', 'raptor_CAN1.dbc','message', 'PM_162','comment', '','signals', {{'PM_motorTemp','PM_rtd4Temp','PM_rtd5Temp','PM_torqueShudder'}},'enabled', [ 1 1 1 1;],'scaled', [ 1 1 1 1;],'canBus', '''CAN1''','messageID', [ 162;],'idMask', [ 536870911;],'payloadMask', [],'payloadValue', [],'period', [ 0;],'mailbox', '''''','queueSize', [ 1;],'label', [ 1;],'ver', [ 2;],'showID', [ 0;],'showRaw', [ 0;],'showRawMsg', [ 0;],'useStartVals', [ 0;],'extendedId', [ 0;],'showAge', [ 1;],'useSimFunc', [ 0;],'sim_func_name', '''''','fill', [ 0;],'editID', [ 0;],'signalOrder', [ 1;],'signalAscDes', [ 1;],'msgLength', [ 8;])  canBus='CAN1'  mailbox=''  payloadMask=[]  payloadValue=[]  idMask=hex2dec('1FFFFFFF')  queueSize=1  showID=0  label=1  fill=0  id=162  showRaw=0  showAge=1  signalOrder=1  signalInfo={{struct('Name', 'PM_torqueShudder','StartBit', [ 48;],'SignalSize', [ 16;],'ByteOrder', 'LittleEndian','ValueType', 'SIGNED','Class', 'int16','Signed', [ 1;],'Factor', [ 0.1;],'Offset', [ 0;],'Min', [ -3276.8;],'Max', [ 3276.7;],'Units', 'Nm','StartVal', [ 0;],'Comment', 'Shudder Compensation Value of Torque','Multiplexed', [ 0;],'Multiplexor', [ 0;],'MultiplexMode_Min', [],'MultiplexMode_Max', []),struct('Name', 'PM_motorTemp','StartBit', [ 32;],'SignalSize', [ 16;],'ByteOrder', 'LittleEndian','ValueType', 'SIGNED','Class', 'int16','Signed', [ 1;],'Factor', [ 0.1;],'Offset', [ 0;],'Min', [ -3276.8;],'Max', [ 3276.7;],'Units', 'degC','StartVal', [ 0;],'Comment', 'Motor Temperature Sensor','Multiplexed', [ 0;],'Multiplexor', [ 0;],'MultiplexMode_Min', [],'MultiplexMode_Max', []),struct('Name', 'PM_rtd5Temp','StartBit', [ 16;],'SignalSize', [ 16;],'ByteOrder', 'LittleEndian','ValueType', 'SIGNED','Class', 'int16','Signed', [ 1;],'Factor', [ 0.1;],'Offset', [ 0;],'Min', [ -3276.8;],'Max', [ 3276.7;],'Units', 'degC','StartVal', [ 0;],'Comment', 'RTD Input 5 (PT1000) Temperature (Gen 2 Only)','Multiplexed', [ 0;],'Multiplexor', [ 0;],'MultiplexMode_Min', [],'MultiplexMode_Max', []),struct('Name', 'PM_rtd4Temp','StartBit', [ 0;],'SignalSize', [ 16;],'ByteOrder', 'LittleEndian','ValueType', 'SIGNED','Class', 'int16','Signed', [ 1;],'Factor', [ 0.1;],'Offset', [ 0;],'Min', [ -3276.8;],'Max', [ 3276.7;],'Units', 'degC','StartVal', [ 0;],'Comment', 'RTD Input 4 (PT1000) Temperature (Gen 2 Only)','Multiplexed', [ 0;],'Multiplexor', [ 0;],'MultiplexMode_Min', [],'MultiplexMode_Max', [])}}  showRawMsg=0  useSimFunc=0  sim_func_name=''  useStartVals=0  extendedId=0
      settings: SourceProductName=Raptor
  raptor_can_rxmsg2 : Raptor_lib/CAN/raptor_can_rxmsg  canDefinition=struct('dbcFile', 'raptor_CAN1.dbc','message', 'PM_160','comment', '','signals', {{'PM_gateDriverBoardTemp','PM_moduleATemp','PM_moduleBTemp','PM_moduleCTemp'}},'enabled', [ 1 1 1 1;],'scaled', [ 1 1 1 1;],'canBus', '''CAN1''','messageID', [ 160;],'idMask', [ 536870911;],'payloadMask', [],'payloadValue', [],'period', [ 0;],'mailbox', '''''','queueSize', [ 1;],'label', [ 1;],'ver', [ 2;],'showID', [ 0;],'showRaw', [ 0;],'showRawMsg', [ 0;],'useStartVals', [ 0;],'extendedId', [ 0;],'showAge', [ 1;],'useSimFunc', [ 0;],'sim_func_name', '''''','fill', [ 0;],'editID', [ 0;],'signalOrder', [ 1;],'signalAscDes', [ 1;],'msgLength', [ 8;])  canBus='CAN1'  mailbox=''  payloadMask=[]  payloadValue=[]  idMask=hex2dec('1FFFFFFF')  queueSize=1  showID=0  label=1  fill=0  id=160  showRaw=0  showAge=1  signalOrder=1  signalInfo={{struct('Name', 'PM_moduleCTemp','StartBit', [ 32;],'SignalSize', [ 16;],'ByteOrder', 'LittleEndian','ValueType', 'SIGNED','Class', 'int16','Signed', [ 1;],'Factor', [ 0.1;],'Offset', [ 0;],'Min', [ 0;],'Max', [ 0;],'Units', 'degC','StartVal', [ 0;],'Comment', 'IGBT Module C Temperature','Multiplexed', [ 0;],'Multiplexor', [ 0;],'MultiplexMode_Min', [],'MultiplexMode_Max', []),struct('Name', 'PM_moduleBTemp','StartBit', [ 16;],'SignalSize', [ 16;],'ByteOrder', 'LittleEndian','ValueType', 'SIGNED','Class', 'int16','Signed', [ 1;],'Factor', [ 0.1;],'Offset', [ 0;],'Min', [ -3276.8;],'Max', [ 3276.7;],'Units', 'degC','StartVal', [ 0;],'Comment', 'IGBT Module B Temperature','Multiplexed', [ 0;],'Multiplexor', [ 0;],'MultiplexMode_Min', [],'MultiplexMode_Max', []),struct('Name', 'PM_gateDriverBoardTemp','StartBit', [ 48;],'SignalSize', [ 16;],'ByteOrder', 'LittleEndian','ValueType', 'SIGNED','Class', 'int16','Signed', [ 1;],'Factor', [ 0.1;],'Offset', [ 0;],'Min', [ 0;],'Max', [ 0;],'Units', 'degC','StartVal', [ 0;],'Comment', 'Gate Driver Board Temperature','Multiplexed', [ 0;],'Multiplexor', [ 0;],'MultiplexMode_Min', [],'MultiplexMode_Max', []),struct('Name', 'PM_moduleATemp','StartBit', [ 0;],'SignalSize', [ 16;],'ByteOrder', 'LittleEndian','ValueType', 'SIGNED','Class', 'int16','Signed', [ 1;],'Factor', [ 0.1;],'Offset', [ 0;],'Min', [ -3276.8;],'Max', [ 3276.7;],'Units', 'degC','StartVal', [ 0;],'Comment', 'IGBT Module A Temperature','Multiplexed', [ 0;],'Multiplexor', [ 0;],'MultiplexMode_Min', [],'MultiplexMode_Max', [])}}  showRawMsg=0  useSimFunc=0  sim_func_name=''  useStartVals=0  extendedId=0
      settings: SourceProductName=Raptor
  IO_CAN1_PM100DX_Bus : Outport
  wires:
  Bus Creator3/1 -> Bus Creator1/1  "IO_CAN1_160_Bus"
  raptor_can_rxmsg2/5 -> Bus Creator3/5  "PM_moduleCTemp"
  raptor_can_rxmsg2/4 -> Bus Creator3/4  "PM_moduleBTemp"
  raptor_can_rxmsg2/3 -> Bus Creator3/3  "PM_moduleATemp"
  raptor_can_rxmsg2/2 -> Bus Creator3/2  "PM_gateDriverBoardTemp"
  raptor_can_rxmsg2/1 -> Bus Creator3/1  "Age"
  Bus Creator2/1 -> Bus Creator1/2  "IO_CAN1_162_Bus"
  raptor_can_rxmsg1/5 -> Bus Creator2/5  "PM_torqueShudder"
  raptor_can_rxmsg1/3 -> Bus Creator2/3  "PM_rtd4Temp"
  raptor_can_rxmsg1/4 -> Bus Creator2/4  "PM_rtd5Temp"
  raptor_can_rxmsg1/2 -> Bus Creator2/2  "PM_motorTemp"
  raptor_can_rxmsg1/1 -> Bus Creator2/1  "Age"
  Bus Creator1/1 -> IO_CAN1_PM100DX_Bus/1  "IO_CAN1_PM100DX_Bus"
  Bus Creator/1 -> Bus Creator1/3  "IO_CAN1_167_Bus"
  raptor_can_rxmsg/5 -> Bus Creator/5  "PM_vbcVqVolt"
  raptor_can_rxmsg/4 -> Bus Creator/4  "PM_vabVdVolt"
  raptor_can_rxmsg/3 -> Bus Creator/3  "PM_outputVolt"
  raptor_can_rxmsg/2 -> Bus Creator/2  "PM_dcBusVolt"
  raptor_can_rxmsg/1 -> Bus Creator/1  "Age"
